simulink model "CB"  (R2015b)
settings: Solver=FixedStepDiscrete  StartTime=0.0  StopTime=inf  FixedStep=cblk_stepSize  RelTol=1e-3
undefined symbols (not defined in the file): cblc_battChargingMode, cblc_deltaSocThreshBalance, cblc_socThreshBalance, cblc_voltThreshBalance
settings Model: Creator=favv5g  LastModifiedBy=nctzv8
settings ConfigSet: Description=OpenECU configuration set for code generation under RTW-EC.
settings SolverCC: PositivePriorityOrder=on
settings DataIOCC: SaveFormat=Array  SignalLoggingSaveFormat=ModelDataLogs
settings OptimizationCC: DefaultParameterBehavior=Inlined  InlineInvariantSignals=on  ExpressionDepthLimit=2147483647  StateBitsets=on  DataBitsets=on  ZeroExternalMemoryAtStartup=off  ZeroInternalMemoryAtStartup=off  NoFixptDivByZeroProtection=on  EfficientFloat2IntCast=on  OptimizeModelRefInitCode=on  LifeSpan=1
settings DebuggingCC: SaveWithParameterizedLinksMsg=none  SignalResolutionControl=TryResolveAllWithWarning  MultiTaskDSMMsg=warning  MultiTaskCondExecSysMsg=none  SingleTaskRateTransMsg=error  CheckMatrixSingularityMsg=warning  VectorMatrixConversionMsg=warning  FcnCallInpInsideContextMsg=UseLocalSettings  SignalLabelMismatchMsg=warning  StateNameClashWarn=warning
settings HardwareCC: ProdBitPerPointer=32  ProdLargestAtomicInteger=Long  ProdLargestAtomicFloat=Double  ProdEndianess=BigEndian  ProdWordSize=32  ProdHWDeviceType=Freescale->32-bit PowerPC  TargetIntDivRoundTo=Zero  TargetEndianess=BigEndian  TargetHWDeviceType=Freescale->32-bit PowerPC  ProdEqTarget=off
settings RTWCC: SystemTargetFile=openecu_ert.tlc  MakeCommand=make_rtw optimized_floating_point=1  TemplateMakefile=openecu_ert_r2015b_64.tmf  Description=OpenECU Platform Target (ERT, optimised floating-point code)  RetainRTWFile=on  IncludeHyperlinkInReport=on
settings CodeAppCC: ForceParamTrailComments=on  IgnoreCustomStorageClasses=off  SimulinkDataObjDesc=on  CustomSymbolStrType=$N$R$M  InsertBlockDesc=on  InternalIdentifier=Classic
settings STFCustomTargetCC: TargetLibSuffix=.a  GenerateSampleERTMain=on  ConcurrentExecutionCompliant=off  IncludeMdlTerminateFcn=off  GeneratePreprocessorConditionals=Use local settings  CombineOutputUpdateFcns=on  IncludeFileDelimiter=UseQuote  ERTCustomFileBanners=on  SupportContinuousTime=off  MATLABClassNameForMDSCustomization=Simulink.SoftwareTarget.ERTCustomization  CPPClassGenCompliant=off  GRTInterface=off  SystemTargetFile=openecu_ert.tlc
settings ERTTargetCC: GenerateSampleERTMain=on  ParMdlRefBuildCompliant=off  CompOptLevelCompliant=off  ConcurrentExecutionCompliant=off  IncludeMdlTerminateFcn=off  ERTFirstTimeCompliant=off  IncludeFileDelimiter=UseQuote  SupportNonInlinedSFcns=on  ModelStepFunctionPrototypeControlCompliant=off  CPPClassGenCompliant=off  UseToolchainInfoCompliant=off  ExtModeMexFile=noextcomm  InlinedParameterPlacement=NonHierarchical  ERTSrcFileBannerTemplate=oe_code_c_template.cgt  ERTHdrFileBannerTemplate=oe_code_h_template.cgt  ERTDataSrcFileTemplate=oe_data_c_template.cgt  ERTDataHdrFileTemplate=oe_data_h_template.cgt  ERTCustomFileTemplate=example_file_process.tlc  GlobalDataDefinition=InSeparateSourceFile  GlobalDataReference=InSeparateHeaderFile  EnableUserReplacementTypes=on

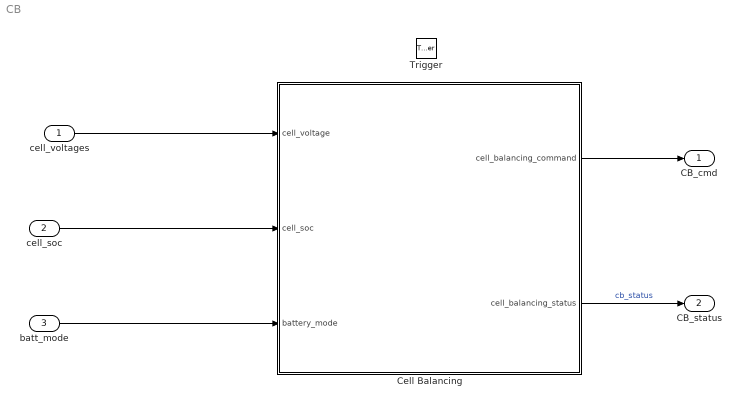
== system CB ==
  cell_voltages : Inport
  cell_soc : Inport  Port=2
  batt_mode : Inport  Port=3  OutDataTypeStr=uint8
  Trigger : TriggerPort  TriggerType=function-call  PortDimensions=1
  Cell Balancing : Subsystem  TreatAsAtomicUnit=on
  CB_cmd : Outport
  CB_status : Outport  Port=2
  wires:
  cell_voltages/1 -> Cell Balancing/1(cell_voltage)
  batt_mode/1 -> Cell Balancing/3(battery_mode)
  cell_soc/1 -> Cell Balancing/2(cell_soc)
  Cell Balancing/1(cell_balancing_command) -> CB_cmd/1
  Cell Balancing/2(cell_balancing_status) -> CB_status/1  "cb_status"

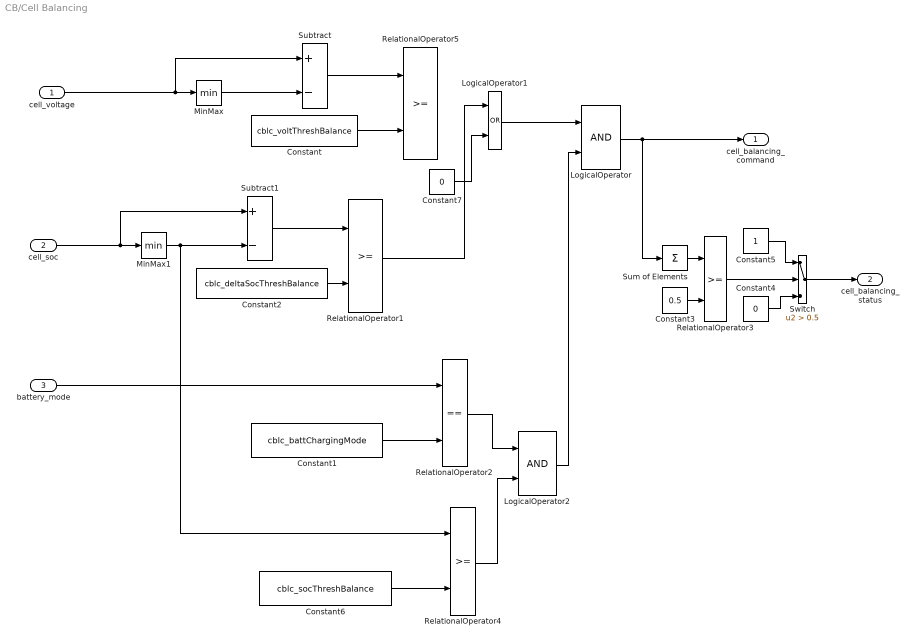
== system CB/Cell Balancing ==
  cell_voltage : Inport  PortDimensions=40
  cell_soc : Inport  Port=2  PortDimensions=40
  battery_mode : Inport  Port=3
  Constant : Constant  Value=cblc_voltThreshBalance
  Constant1 : Constant  Value=cblc_battChargingMode
  Constant2 : Constant  Value=cblc_deltaSocThreshBalance
  Constant3 : Constant  Value=0.5
  Constant4 : Constant  Value=0  OutDataTypeStr=boolean
  Constant5 : Constant  OutDataTypeStr=boolean
  Constant6 : Constant  Value=cblc_socThreshBalance
  Constant7 : Constant  Value=0
  LogicalOperator : Logic  AllPortsSameDT=off  OutDataTypeStr=boolean
  LogicalOperator1 : Logic  Operator=OR  AllPortsSameDT=off  OutDataTypeStr=boolean
  LogicalOperator2 : Logic  AllPortsSameDT=off  OutDataTypeStr=boolean
  MinMax : MinMax
  MinMax1 : MinMax
  RelationalOperator{1,3..5} (4 alike) : RelationalOperator  OutDataTypeStr=boolean
  RelationalOperator2 : RelationalOperator  Operator===  OutDataTypeStr=boolean
  Subtract : Sum  Inputs=+-
  Subtract1 : Sum  Inputs=+-
  Sum of Elements : Sum  Inputs=+
  Switch : Switch  Criteria=u2 > Threshold  Threshold=0.5
  cell_balancing_command : Outport
  cell_balancing_status : Outport  Port=2
  wires:
  Subtract/1 -> RelationalOperator5/1
  Constant/1 -> RelationalOperator5/2
  cell_voltage/1 -> Subtract/1, MinMax/1
  MinMax/1 -> Subtract/2
  battery_mode/1 -> RelationalOperator2/1
  Constant1/1 -> RelationalOperator2/2
  Subtract1/1 -> RelationalOperator1/1
  Constant2/1 -> RelationalOperator1/2
  cell_soc/1 -> Subtract1/1, MinMax1/1
  MinMax1/1 -> RelationalOperator4/1, Subtract1/2
  LogicalOperator1/1 -> LogicalOperator/1
  LogicalOperator/1 -> cell_balancing_command/1, Sum of Elements/1
  Sum of Elements/1 -> RelationalOperator3/1
  Constant3/1 -> RelationalOperator3/2
  RelationalOperator3/1 -> Switch/2
  Constant4/1 -> Switch/3
  Constant5/1 -> Switch/1
  Switch/1 -> cell_balancing_status/1
  Constant6/1 -> RelationalOperator4/2
  RelationalOperator2/1 -> LogicalOperator2/1
  RelationalOperator4/1 -> LogicalOperator2/2
  LogicalOperator2/1 -> LogicalOperator/2
  Constant7/1 -> LogicalOperator1/2
  RelationalOperator1/1 -> LogicalOperator1/1
